simulink model "w1que2"  (R2020b)
settings: Solver=VariableStepAuto  StartTime=0.0  StopTime=10.0  RelTol=1e-3
settings Model: Creator=ANUJA  LastModifiedBy=ANUJA

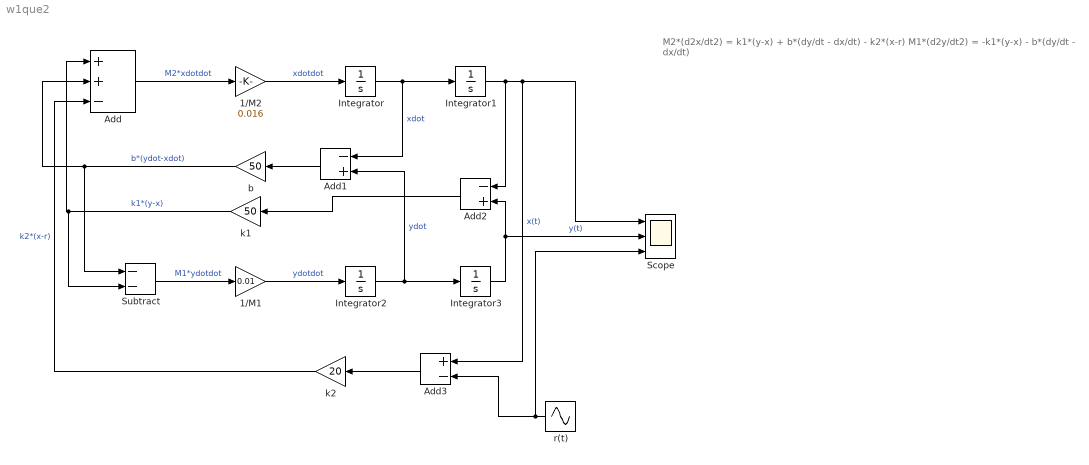
== system w1que2 ==
  note: M2*(d2x/dt2) = k1*(y-x) + b*(dy/dt - dx/dt) - k2*(x-r)
      |
      | M1*(d2y/dt2) = -k1*(y-x) - b*(dy/dt - dx/dt)
  1/M1 : Gain  Gain=0.01
  1/M2 : Gain  Gain=0.016
  Add : Sum  Inputs=++-
  Add1 : Sum  Inputs=-+
  Add2 : Sum  Inputs=-+
  Add3 : Sum  Inputs=+-
  Integrator{,1..3} (4 alike) : Integrator
  Scope : Scope  NumInputPorts=3
  Subtract : Sum  Inputs=--
  b : Gain  Gain=50
  k1 : Gain  Gain=50
  k2 : Gain  Gain=20
  r(t) : Sin  Amplitude=2  SampleTime=0
  wires:
  Add3/1 -> k2/1
  k2/1 -> Add/3  "k2*(x-r)"
  Subtract/1 -> 1/M1/1  "M1*ydotdot"
  Integrator/1 -> Add1/1, Integrator1/1  "xdot"
  Add1/1 -> b/1
  b/1 -> Subtract/1, Add/2  "b*(ydot-xdot)"
  r(t)/1 -> Scope/3, Add3/2
  Integrator2/1 -> Integrator3/1, Add1/2  "ydot"
  Integrator1/1 -> Add3/1, Scope/1, Add2/1  "x(t)"
  Add/1 -> 1/M2/1  "M2*xdotdot"
  Add2/1 -> k1/1
  k1/1 -> Subtract/2, Add/1  "k1*(y-x)"
  1/M1/1 -> Integrator2/1  "ydotdot"
  1/M2/1 -> Integrator/1  "xdotdot"
  Integrator3/1 -> Add2/2, Scope/2  "y(t)"
